simulink model "Model_daq"  (R2018b)
settings: Solver=ode3  StartTime=0.0  StopTime=10  FixedStep=0.02  MaxStep=0.02  RelTol=1e-3
values from neighbouring files (symbols this model uses):
  denH = [0.1 1]    [definitivo.mat]
  Fmax = 200    [Project.m]    (also in definitivo.mat)
  m_load = 10    [Project.m]    (also in definitivo.mat; robot_dynamics.m = d(3))
  numH = [100 100]    [definitivo.mat]
  Ts = 1/fs    (= 0.02)    [Project.m]    (also in definitivo.mat)
libraries: simulink x3
settings Model: Creator=Andrea Ghezzi  LastModifiedBy=sl65b
settings OptimizationCC: BlockReduction=off  DefaultParameterBehavior=Inlined  BufferReuse=off

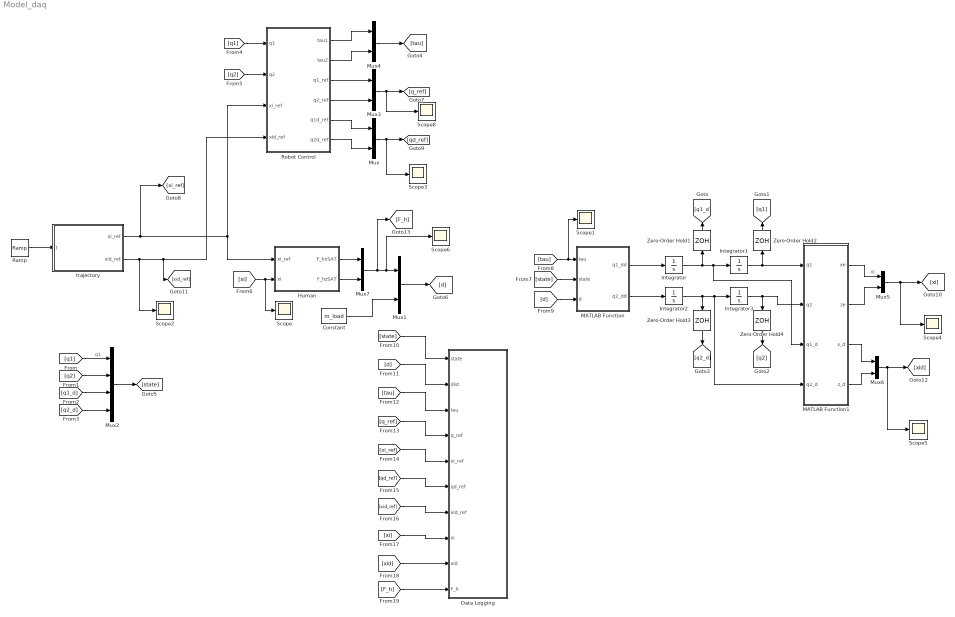
== system Model_daq ==
  Constant : Constant  Value=m_load
  Data Logging : Subsystem
  "Human " : Subsystem
  Integrator : Integrator
  Integrator1 : Integrator  InitialCondition=2.18
  Integrator2 : Integrator
  Integrator3 : Integrator  InitialCondition=2.72
  MATLAB Function : MATLAB Function  TreatAsAtomicUnit=on
  MATLAB Function1 : MATLAB Function  TreatAsAtomicUnit=on
  Mux{,1,3..7} (7 alike) : Mux  Inputs=2
  Mux2 : Mux
  Ramp : simulink/Sources/Ramp  slope=1  start=0  InitialOutput=0
  Robot Control : Subsystem
  Scope{,1..6,8} (8 alike) : Scope
  Zero-Order Hold{1..4} (4 alike) : ZeroOrderHold  SampleTime=Ts
  trajectory : MATLAB Function  TreatAsAtomicUnit=on
  wires:
  Ramp/1 -> trajectory/1("t ")
  trajectory/1(xi_ref) -> "Human "/1(xi_ref), Robot Control/3(xi_ref), [xi_ref]
  Constant/1 -> Mux1/2
  [q1] -> Mux2/1  "q1"
  [q2] -> Mux2/2
  [q1_d] -> Mux2/3
  [q2_d] -> Mux2/4
  [xi] -> Scope/1, "Human "/2(xi)
  [q1] -> Robot Control/1(q1)
  [q2] -> Robot Control/2(q2)
  Mux2/1 -> [state]
  [state] -> MATLAB Function/2(state)
  Integrator2/1 -> MATLAB Function1/4(q2_d), Integrator3/1, Zero-Order Hold3/1
  Integrator1/1 -> MATLAB Function1/1(q1), Zero-Order Hold2/1
  Integrator3/1 -> MATLAB Function1/2(q2), Zero-Order Hold4/1
  Zero-Order Hold1/1 -> [q1_d]
  Zero-Order Hold3/1 -> [q2_d]
  Zero-Order Hold2/1 -> [q1]
  Zero-Order Hold4/1 -> [q2]
  Integrator/1 -> MATLAB Function1/3(q1_d), Integrator1/1, Zero-Order Hold1/1
  MATLAB Function/1(q1_dd) -> Integrator/1
  MATLAB Function/2(q2_dd) -> Integrator2/1
  Mux1/1 -> [d]
  Mux3/1 -> Scope8/1, [q_ref]
  Robot Control/4(q2_ref) -> Mux3/2
  Robot Control/3("q1_ref ") -> Mux3/1
  [state] -> Data Logging/1(state)
  [d] -> Data Logging/2(dist)
  [tau] -> Data Logging/3(tau)
  [q_ref] -> Data Logging/4("q_ref ")
  Robot Control/1(tau1) -> Mux4/1
  Robot Control/2(tau2) -> Mux4/2
  Mux4/1 -> [tau]
  [tau] -> Scope1/1, MATLAB Function/1(tau)
  [xi_ref] -> Data Logging/5(xi_ref)
  [d] -> MATLAB Function/3(d)
  Robot Control/5(q1d_ref) -> Mux/1
  Robot Control/6(q2d_ref) -> Mux/2
  Mux/1 -> Scope3/1, [qd_ref]
  [qd_ref] -> Data Logging/6("qd_ref ")
  trajectory/2(xid_ref) -> Scope2/1, [xid_ref], Robot Control/4(xid_ref)
  [xid_ref] -> Data Logging/7(xid_ref)
  MATLAB Function1/1(xe) -> Mux5/1  "xi"
  MATLAB Function1/2(ze) -> Mux5/2
  Mux5/1 -> Scope4/1, [xi]
  MATLAB Function1/3(x_d) -> Mux6/1
  MATLAB Function1/4(z_d) -> Mux6/2
  Mux6/1 -> Scope5/1, [xid]
  [xi] -> Data Logging/8("xi ")
  [xid] -> Data Logging/9(xid)
  [F_h] -> Data Logging/10("F_h ")
  Mux7/1 -> [F_h], Scope6/1, Mux1/1
  "Human "/2(F_hzSAT) -> Mux7/2
  "Human "/1(F_hxSAT) -> Mux7/1

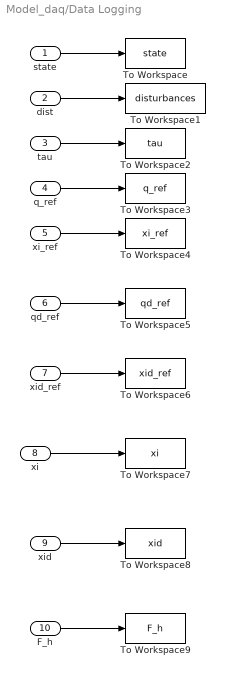
== system Model_daq/Data Logging ==
  state : Inport
  dist : Inport  Port=2
  tau : Inport  Port=3
  "q_ref " : Inport  Port=4
  xi_ref : Inport  Port=5
  "qd_ref " : Inport  Port=6
  xid_ref : Inport  Port=7
  "xi " : Inport  Port=8
  xid : Inport  Port=9
  "F_h " : Inport  Port=10
  To Workspace : ToWorkspace  VariableName=state  SampleTime=-1
  To Workspace1 : ToWorkspace  VariableName=disturbances  SampleTime=-1
  To Workspace2 : ToWorkspace  VariableName=tau  SampleTime=-1
  To Workspace3 : ToWorkspace  VariableName=q_ref  SampleTime=-1
  To Workspace4 : ToWorkspace  VariableName=xi_ref  SampleTime=-1
      settings: Save2DSignal=2-D array (concatenate along first dimension)
  To Workspace5 : ToWorkspace  VariableName=qd_ref  SampleTime=-1
      settings: Save2DSignal=2-D array (concatenate along first dimension)
  To Workspace6 : ToWorkspace  VariableName=xid_ref  SampleTime=-1
      settings: Save2DSignal=2-D array (concatenate along first dimension)
  To Workspace7 : ToWorkspace  VariableName=xi  SampleTime=-1
      settings: Save2DSignal=2-D array (concatenate along first dimension)
  To Workspace8 : ToWorkspace  VariableName=xid  SampleTime=-1
      settings: Save2DSignal=2-D array (concatenate along first dimension)
  To Workspace9 : ToWorkspace  VariableName=F_h  SampleTime=-1
  wires:
  state/1 -> To Workspace/1
  dist/1 -> To Workspace1/1
  tau/1 -> To Workspace2/1
  "q_ref "/1 -> To Workspace3/1
  xi_ref/1 -> To Workspace4/1
  "qd_ref "/1 -> To Workspace5/1
  xid_ref/1 -> To Workspace6/1
  "xi "/1 -> To Workspace7/1
  xid/1 -> To Workspace8/1
  "F_h "/1 -> To Workspace9/1

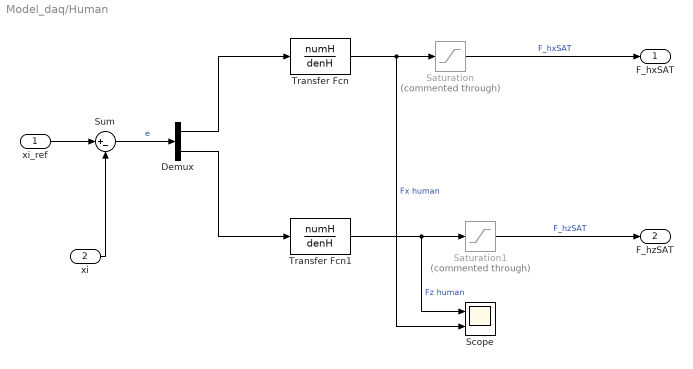
== system Model_daq/Human  ==
  xi_ref : Inport
  xi : Inport  Port=2
  Demux : Demux  Outputs=2
  Saturation : Saturate  Commented=through  UpperLimit=Fmax  LowerLimit=-Fmax
  Saturation1 : Saturate  Commented=through  UpperLimit=Fmax  LowerLimit=-Fmax
  Scope : Scope  NumInputPorts=2
  Sum : Sum  Inputs=|+-
  Transfer Fcn : TransferFcn  Numerator=numH  Denominator=denH
  Transfer Fcn1 : TransferFcn  Numerator=numH  Denominator=denH
  F_hxSAT : Outport
  F_hzSAT : Outport  Port=2
  wires:
  Transfer Fcn/1 -> Scope/2, Saturation/1  "Fx human"
  Sum/1 -> Demux/1  "e"
  Transfer Fcn1/1 -> Scope/1, Saturation1/1  "Fz human"
  xi/1 -> Sum/2
  xi_ref/1 -> Sum/1
  Saturation/1 -> F_hxSAT/1  "F_hxSAT"
  Saturation1/1 -> F_hzSAT/1  "F_hzSAT"
  Demux/1 -> Transfer Fcn/1
  Demux/2 -> Transfer Fcn1/1

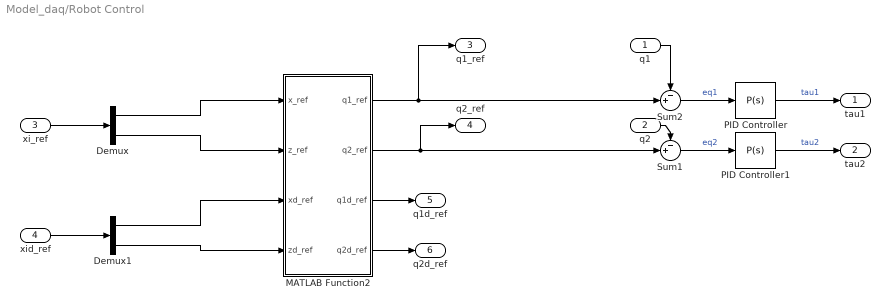
== system Model_daq/Robot Control ==
  q1 : Inport
  q2 : Inport  Port=2
  xi_ref : Inport  Port=3
  xid_ref : Inport  Port=4
  Demux : Demux  Outputs=2
  Demux1 : Demux  Outputs=2
  MATLAB Function2 : MATLAB Function  TreatAsAtomicUnit=on
  PID Controller : simulink/Continuous/PID Controller  Controller=P  Form=Parallel  TimeDomain=Continuous-time  SampleTime=-1  IntegratorMethod=Forward Euler  FilterMethod=Forward Euler  ControllerParametersSource=internal  P=0  I=1096.09901966968  D=513.581840866343  UseFilter=on  N=626.306180697594  TunerSelectOption=Transfer Function Based (PID Tuner App)  InitialConditionSource=internal  InitialConditionForIntegrator=0  InitialConditionForFilter=0  DifferentiatorICPrevScaledInput=0  ExternalReset=none  TrackingMode=off  Kt=1  LimitOutput=off  UpperSaturationLimit=inf  LowerSaturationLimit=-inf  LinearizeAsGain=on  AntiWindupMode=none  Kb=1  POutMin=[]  POutMax=[]  IOutMin=[]  IOutMax=[]  DOutMin=[]  DOutMax=[]  NOutMin=[]  NOutMax=[]  SumOutMin=[]  SumOutMax=[]  SaturationOutMin=[]  SaturationOutMax=[]  PParamMin=[]  PParamMax=[]  IParamMin=[]  IParamMax=[]  DParamMin=[]  DParamMax=[]  NParamMin=[]  NParamMax=[]  KbParamMin=[]  KbParamMax=[]  KtParamMin=[]  KtParamMax=[]  KbOutMin=[]  KbOutMax=[]  KtOutMin=[]  KtOutMax=[]  IntegratorOutMin=[]  IntegratorOutMax=[]  FilterOutMin=[]  FilterOutMax=[]  SumI1OutMin=[]  SumI1OutMax=[]  SumI2OutMin=[]  SumI2OutMax=[]  SumI3OutMin=[]  SumI3OutMax=[]  SumI4OutMin=[]  SumI4OutMax=[]  SumDOutMin=[]  SumDOutMax=[]  DifferentiatorOutMin=[]  DifferentiatorOutMax=[]  FilterDiffOutCoefMin=[]  FilterDiffOutCoefMax=[]  ReciprocalOutMin=[]  ReciprocalOutMax=[]  SumDenOutMin=[]  SumDenOutMax=[]  SumNumOutMin=[]  SumNumOutMax=[]  DivideOutMin=[]  DivideOutMax=[]  IntegratorContinuousStateAttributes=''  IntegratorStateMustResolveToSignalObject=off  IntegratorRTWStateStorageClass=Auto  FilterContinuousStateAttributes=''  FilterStateMustResolveToSignalObject=off  FilterRTWStateStorageClass=Auto  ParallelPVariant=InternalParameters  IdealPVariant=Disabled  IVariant=Disabled  DVariant=Disabled  IntegratorVariant=Disabled  SatVariant=Disabled  AWVariant=Disabled  PCopyVariant=Disabled  TRVariant=Disabled  FdbkBlocksVariant=Forward  IdealPFdbkVariant=Disabled  SatFdbkVariant=Disabled  DerivativeFilterVariant=Disabled  NVariant=Disabled  NCopyVariant=Disabled_SignalSpec  FilterICVariant=Disabled  IntegratorICVariant=Disabled  ExternalResetVariant=Disabled  TRSumVariant=Passthrough  SumFdbkVariant=Disabled  SumVariant=Passthrough_P
  PID Controller1 : simulink/Continuous/PID Controller  Controller=P  Form=Parallel  TimeDomain=Continuous-time  SampleTime=-1  IntegratorMethod=Forward Euler  FilterMethod=Forward Euler  ControllerParametersSource=internal  P=0  I=1  D=1  UseFilter=on  N=854.342384892563  TunerSelectOption=Transfer Function Based (PID Tuner App)  InitialConditionSource=internal  InitialConditionForIntegrator=0  InitialConditionForFilter=0  DifferentiatorICPrevScaledInput=0  ExternalReset=none  TrackingMode=off  Kt=1  LimitOutput=off  UpperSaturationLimit=inf  LowerSaturationLimit=-inf  LinearizeAsGain=on  AntiWindupMode=none  Kb=1  POutMin=[]  POutMax=[]  IOutMin=[]  IOutMax=[]  DOutMin=[]  DOutMax=[]  NOutMin=[]  NOutMax=[]  SumOutMin=[]  SumOutMax=[]  SaturationOutMin=[]  SaturationOutMax=[]  PParamMin=[]  PParamMax=[]  IParamMin=[]  IParamMax=[]  DParamMin=[]  DParamMax=[]  NParamMin=[]  NParamMax=[]  KbParamMin=[]  KbParamMax=[]  KtParamMin=[]  KtParamMax=[]  KbOutMin=[]  KbOutMax=[]  KtOutMin=[]  KtOutMax=[]  IntegratorOutMin=[]  IntegratorOutMax=[]  FilterOutMin=[]  FilterOutMax=[]  SumI1OutMin=[]  SumI1OutMax=[]  SumI2OutMin=[]  SumI2OutMax=[]  SumI3OutMin=[]  SumI3OutMax=[]  SumI4OutMin=[]  SumI4OutMax=[]  SumDOutMin=[]  SumDOutMax=[]  DifferentiatorOutMin=[]  DifferentiatorOutMax=[]  FilterDiffOutCoefMin=[]  FilterDiffOutCoefMax=[]  ReciprocalOutMin=[]  ReciprocalOutMax=[]  SumDenOutMin=[]  SumDenOutMax=[]  SumNumOutMin=[]  SumNumOutMax=[]  DivideOutMin=[]  DivideOutMax=[]  IntegratorContinuousStateAttributes=''  IntegratorStateMustResolveToSignalObject=off  IntegratorRTWStateStorageClass=Auto  FilterContinuousStateAttributes=''  FilterStateMustResolveToSignalObject=off  FilterRTWStateStorageClass=Auto  ParallelPVariant=InternalParameters  IdealPVariant=Disabled  IVariant=Disabled  DVariant=Disabled  IntegratorVariant=Disabled  SatVariant=Disabled  AWVariant=Disabled  PCopyVariant=Disabled  TRVariant=Disabled  FdbkBlocksVariant=Forward  IdealPFdbkVariant=Disabled  SatFdbkVariant=Disabled  DerivativeFilterVariant=Disabled  NVariant=Disabled  NCopyVariant=Disabled_SignalSpec  FilterICVariant=Disabled  IntegratorICVariant=Disabled  ExternalResetVariant=Disabled  TRSumVariant=Passthrough  SumFdbkVariant=Disabled  SumVariant=Passthrough_P
  Sum1 : Sum  Inputs=-+|
  Sum2 : Sum  Inputs=-+|
  tau1 : Outport
  tau2 : Outport  Port=2
  "q1_ref " : Outport  Port=3
  q2_ref : Outport  Port=4
  q1d_ref : Outport  Port=5
  q2d_ref : Outport  Port=6
  wires:
  MATLAB Function2/1(q1_ref) -> "q1_ref "/1, Sum2/2
  Demux/1 -> MATLAB Function2/1(x_ref)
  PID Controller1/1 -> tau2/1  "tau2"
  PID Controller/1 -> tau1/1  "tau1"
  q1/1 -> Sum2/1
  Sum1/1 -> PID Controller1/1  "eq2"
  Demux/2 -> MATLAB Function2/2(z_ref)
  Sum2/1 -> PID Controller/1  "eq1"
  MATLAB Function2/2(q2_ref) -> Sum1/2, q2_ref/1
  xi_ref/1 -> Demux/1
  q2/1 -> Sum1/1
  MATLAB Function2/3(q1d_ref) -> q1d_ref/1
  MATLAB Function2/4(q2d_ref) -> q2d_ref/1
  Demux1/1 -> MATLAB Function2/3(xd_ref)
  Demux1/2 -> MATLAB Function2/4(zd_ref)
  xid_ref/1 -> Demux1/1

== matlab function Model_daq/trajectory ==
  data: xi_ref output; t input; xid_ref output
function [xi_ref, xid_ref] = trajectory(t)
t0 = 0;
tf = 4;
pos_0 = [0 0];
pos_f = [1 1];
vel_0 = [0 0];
vel_f = [0 0];
T = tf-t0;

if t<4
    a0 = pos_0;
    a1 = vel_0;
    a2 = (-3*(pos_0-pos_f)-(2*vel_0+vel_f)*T)/T^2;
    a3 = (2*(pos_0-pos_f)+(vel_0+vel_f)*T)/T^3;
    xi_ref = a0+a1*(t-t0)+a2*(t-t0)^2+a3*(t-t0)^3;    %positions
    xid_ref = a1+2*a2*(t-t0)+3*a3*(t-t0)^2;           %speeds
    acc = 2*a2+6*a3*(t-t0);                           %accelerations          
else
    xi_ref = pos_f;
    xid_ref = [0 0];
    acc = [0 0];
   
end

== matlab function Model_daq/MATLAB Function ==
  data: tau input; q1_dd output; state input; d input; q2_dd output
function [q1_dd, q2_dd] = robot_dynamics(tau, state, d)

F_hx = d(1);
F_hz = d(2);
m_load = d(3);
q1  = state(1);
q2 = state(2);
q1_d = state(3);
q2_d = state(4); 

%robot parameters
g   = 9.81;
J1  = 10;   %inertia link 1
J2  = 10;   %inertia link 2
m1  = 50;   %mass link 1
m2  = 50;   %mass link 2
a1  = 1.2;    %lenght link 1
a2  = 1;  %length link 2
ac1  = a1/2; %centre of mass link 1
ac2  = a2/2; %centre of mass link 2

%kinematic functions
% q1          = q(1);
% q2          = q(2);
% q1_d        = q_d(1);
% q2_d        = q_d(2);
c1          = cos(q1);
s1          = sin(q1);
c2          = cos(q2);
s2          = sin(q2);
c12         = cos(q1+q2);
s12         = sin(q1+q2);

J        = [-a1*sin(q1)-a2*sin(q1+q2)  -a2*sin(q1+q2);
             a1*cos(q1)+a2*cos(q1+q2)   a2*cos(q1+q2)];
         
M_tot =  [m1*ac1^2+m2*(a1^2+ac2^2+2*a1*ac2*c2)+J1+J2     m2*(ac2^2+a1*ac2*c2)+J2;
              m2*(ac2^2+a1*ac2*c2)+J2                    m2*ac2^2+J2];
              
% C_tot = [-a1*q2_d*s2*ac2*m2   -a1*q1_d*s2*ac2*m2;
%           -a1*q1_d*s2*ac2*m2             0];
%- C_tot*[q1_d;q2_d]
         
g_tot = [(m1*ac1+m2*a1)*g*c1+m2*g*ac2*c12;
                 m2*g*ac2*c12];


 %equation of motion of the 2dof manipulator 
q_dd = inv(M_tot)*(tau + J'*[F_hx;F_hz - m_load*g] - g_tot);
q1_dd = q_dd(1);
q2_dd = q_dd(2);
 
end

== matlab function Model_daq/Robot Control/MATLAB Function2 ==
  data: x_ref input; q1_ref output; z_ref input; q2_ref output; xd_ref input; zd_ref input; q1d_ref output; q2d_ref output
function [q1_ref, q2_ref, q1d_ref, q2d_ref] = inverse_kin(x_ref, z_ref, xd_ref, zd_ref)

%robot parameters
a1  = 1.2;    %lenght link 1
a2  = 1;  %length link 2

%moving the robot half meter right from the origin
%DOING SO WE DON'T HAVE ANY KINEMATIC SINGULARITIES
%% computation of positions
x_ref=x_ref-0.5;
c2 = (x_ref^2+z_ref^2-a1^2-a2^2)/(2*a1*a2);
s2 = sqrt(1-c2^2);
q2_ref = atan2(s2,c2);
q1_ref = atan2(z_ref,x_ref)-atan2(a2*s2, a1+a2*c2);

%% computation of reference joints speeds

J        = [-a1*sin(q1_ref)-a2*sin(q1_ref+q2_ref)  -a2*sin(q1_ref+q2_ref);
             a1*cos(q1_ref)+a2*cos(q1_ref+q2_ref)   a2*cos(q1_ref+q2_ref)];
         
qd_ref = J\[xd_ref;zd_ref];
q1d_ref = qd_ref(1,1);
q2d_ref = qd_ref(2,1);

end

== matlab function Model_daq/MATLAB Function1 ==
  data: q1 input; xe output; q2 input; q1_d input; q2_d input; ze output; x_d output; z_d output
function [xe, ze, x_d, z_d]   = direct_kin_test(q1, q2, q1_d, q2_d)
%robot parameters
a1  = 1.2;    %lenght link 1
a2  = 1;  %length link 2

%kinematic functions
c1= cos(q1);
s1= sin(q1);
c2= cos(q2);
s2= sin(q2);
c12= cos(q1+q2);
s12= sin(q1+q2);

% Computation of end effector quantities given the measure joints
% quantities
if q1 == 0 && q2 == 0
    xe = 0;
    ze = 0;
   
else 
    xe = 0.5 + a1*c1 + a2*c12;
    ze = a1*s1 + a2*s12;
    
end
%xi = [xe;ze];
    
%% computations of speeds
J        = [-a1*sin(q1)-a2*sin(q1+q2)  -a2*sin(q1+q2);
             a1*cos(q1)+a2*cos(q1+q2)   a2*cos(q1+q2)];

xi_d = J*[q1_d;q2_d];

x_d = xi_d(1,1);
z_d = xi_d(2,1);
   
end
